simulink model "Model_simulink_dyskretny_impact_torque_NO_QUANTIZER"  (R2017a)
settings: Solver=ode45  StartTime=0.0  StopTime=Tend  FixedStep=Tp  RelTol=1e-3
values from neighbouring files (symbols this model uses):
  In = 130.7    [Skrypt_do_schematu.m]
  J = Js+Jmr    (= 5.82)    [Skrypt_do_schematu.m]
  K1 = Kw    [Skrypt_do_schematu.m]
  K2 = Kw*(Tp/TR-1)    [Skrypt_do_schematu.m]
  K3 = m/V    [Skrypt_do_schematu.m]
  K4 = (Tp-m)/V    [Skrypt_do_schematu.m]
  Kp = 0.15*Un    (= 66)    [Skrypt_do_schematu.m]
  Kt = 10/(1.2*wn)    (= 0.0548810148593)    [Skrypt_do_schematu.m]
  Lambda = 2    [Skrypt_do_schematu.m]
  Mn = psi * In    (= 350.156554572)    [Skrypt_do_schematu.m]
  psi = (Un-(Rt*In))/wn    (= 2.67908610996)    [Skrypt_do_schematu.m]
  Rt = 0.254    [Skrypt_do_schematu.m]
  T = Lt/Rt    (= 0.00641732283465)    [Skrypt_do_schematu.m]
  Tp = Beta/N    (= 0.002)    [Skrypt_do_schematu.m]
  Un = 440    [Skrypt_do_schematu.m]
  Uz0 = (Lambda*In)*((Y*B1)/(B1-Beta))    [Skrypt_do_schematu.m]
  wn = (2*pi*n)/60    (= 151.843644924)    [Skrypt_do_schematu.m]
  Y = 7.8/(2.5*In)    (= 0.0238714613619)    [Skrypt_do_schematu.m]
settings Model: Creator=user  LastModifiedBy=a
settings DataIOCC: LimitDataPoints=on  SaveFormat=Array  SignalLoggingSaveFormat=ModelDataLogs
settings OptimizationCC: BlockReduction=off  BooleanDataType=off  ExpressionDepthLimit=2147483647  LifeSpan=inf
settings DebuggingCC: SaveWithParameterizedLinksMsg=none  UnderspecifiedInitializationDetection=Classic  MergeDetectMultiDrivingBlocksExec=none  SignalResolutionControl=TryResolveAllWithWarning  MultiTaskDSMMsg=warning  MultiTaskCondExecSysMsg=none  StateNameClashWarn=warning  SFUnexpectedBacktrackingDiag=warning  SFNoUnconditionalDefaultTransitionDiag=warning  SFExecutionAtInitializationDiag=none
settings HardwareCC: ProdBitPerPointer=32  ProdBitPerSizeT=32  ProdBitPerPtrDiffT=32  ProdLargestAtomicFloat=None  ProdIntDivRoundTo=Undefined  ProdEndianess=Unspecified  ProdWordSize=32  ProdHWDeviceType=32-bit Generic  TargetUnknown=on
settings ModelReferenceCC: PropagateSignalLabelsOutOfModel=off
settings GRTTargetCC: TargetLangStandard=C89/C90 (ANSI)  GeneratePreprocessorConditionals=Disable all
settings ConfigComp: CovMetricSettings=dw  CovHtmlReporting=on  CovSaveCumulativeToWorkspaceVar=on  CovSaveSingleToWorkspaceVar=on  CovExternalEMLEnable=off

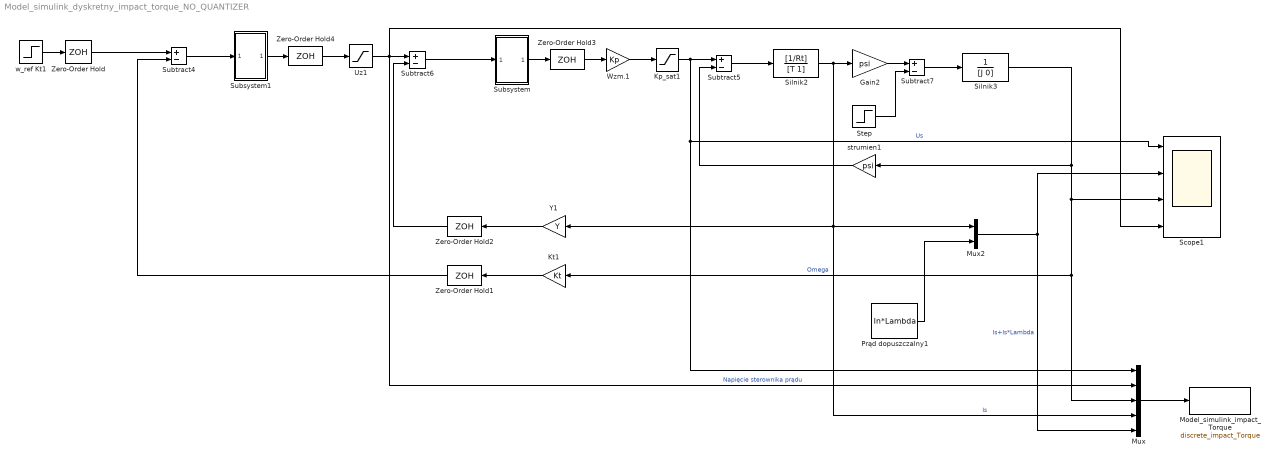
== system Model_simulink_dyskretny_impact_torque_NO_QUANTIZER ==
  Gain2 : Gain  Gain=psi
  Kp_sat1 : Saturate  UpperLimit=1.5*Un  LowerLimit=-1.5*Un
  Kt1 : Gain  Gain=Kt
  Model_simulink_impact_Torque : ToWorkspace  VariableName=discrete_impact_Torque  SaveFormat=Structure With Time  SampleTime=Tp
  Mux : Mux  Inputs=5
  Mux2 : Mux  Inputs=2
  Prąd dopuszczalny1 : Constant  Value=In*Lambda
  Scope1 : Scope  NumInputPorts=4
  Silnik2 : TransferFcn  Numerator=[1/Rt]  Denominator=[T 1]
  Silnik3 : TransferFcn  Numerator=1  Denominator=[J 0]
  Step : Step  Time=5  After=Mn  SampleTime=0
  Subsystem : Subsystem
  Subsystem1 : Subsystem
  Subtract{4..7} (4 alike) : Sum  Inputs=+-
  Uz1 : Saturate  UpperLimit=Uz0  LowerLimit=-Uz0  SampleTime=Tp
  Wzm.1 : Gain  Gain=Kp
  Y1 : Gain  Gain=Y
  Zero-Order Hold{,1..4} (5 alike) : ZeroOrderHold  SampleTime=Tp
  strumien1 : Gain  Gain=psi
  w_ref Kt1 : Step  Time=0  After=wn*Kt
  wires:
  w_ref Kt1/1 -> Zero-Order Hold/1
  Wzm.1/1 -> Kp_sat1/1
  Subtract5/1 -> Silnik2/1
  Silnik2/1 -> Mux/4, Y1/1, Mux2/1, Gain2/1  "Is"
  Gain2/1 -> Subtract7/1
  Subtract7/1 -> Silnik3/1
  strumien1/1 -> Subtract5/2
  Kp_sat1/1 -> Mux/1, Scope1/1, Subtract5/1  "Us"
  Y1/1 -> Zero-Order Hold2/1
  Mux2/1 -> Mux/5, Scope1/2  "Is+Is*Lambda"
  Prąd dopuszczalny1/1 -> Mux2/2
  Uz1/1 -> Mux/2, Scope1/4, Subtract6/1  "Napięcie sterownika prądu"
  Silnik3/1 -> Mux/3, Kt1/1, Scope1/3, strumien1/1  "Omega"
  Kt1/1 -> Zero-Order Hold1/1
  Step/1 -> Subtract7/2
  Mux/1 -> Model_simulink_impact_Torque/1
  Subtract6/1 -> Subsystem/1(In1)
  Subsystem1/1(Out1) -> Zero-Order Hold4/1
  Subtract4/1 -> Subsystem1/1(In1)
  Zero-Order Hold/1 -> Subtract4/1
  Zero-Order Hold2/1 -> Subtract6/2
  Zero-Order Hold1/1 -> Subtract4/2
  Zero-Order Hold3/1 -> Wzm.1/1
  Subsystem/1(Out1) -> Zero-Order Hold3/1
  Zero-Order Hold4/1 -> Uz1/1

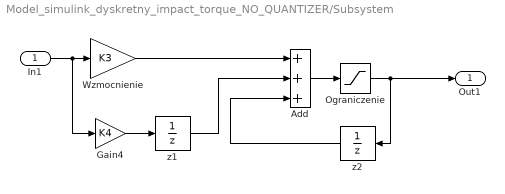
== system Model_simulink_dyskretny_impact_torque_NO_QUANTIZER/Subsystem ==
  In1 : Inport
  Add : Sum  Inputs=+++
  Gain4 : Gain  Gain=K4  SampleTime=Tp
  Ograniczenie : Saturate  UpperLimit=10  LowerLimit=-10
  Wzmocnienie : Gain  Gain=K3  SampleTime=Tp
  z1 : UnitDelay  SampleTime=Tp
  z2 : UnitDelay  SampleTime=Tp
  Out1 : Outport
  wires:
  In1/1 -> Gain4/1, Wzmocnienie/1
  Wzmocnienie/1 -> Add/1
  Gain4/1 -> z1/1
  z1/1 -> Add/2
  Add/1 -> Ograniczenie/1
  Ograniczenie/1 -> Out1/1, z2/1
  z2/1 -> Add/3

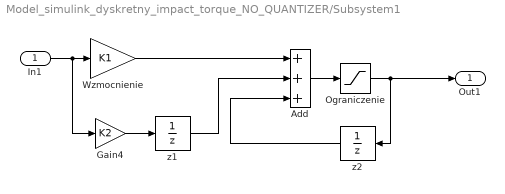
== system Model_simulink_dyskretny_impact_torque_NO_QUANTIZER/Subsystem1 ==
  In1 : Inport
  Add : Sum  Inputs=+++  SampleTime=Tp
  Gain4 : Gain  Gain=K2  SampleTime=Tp
  Ograniczenie : Saturate  UpperLimit=10  LowerLimit=-10
  Wzmocnienie : Gain  Gain=K1  SampleTime=Tp
  z1 : UnitDelay  SampleTime=Tp
  z2 : UnitDelay  SampleTime=Tp
  Out1 : Outport
  wires:
  In1/1 -> Gain4/1, Wzmocnienie/1
  Wzmocnienie/1 -> Add/1
  Gain4/1 -> z1/1
  z1/1 -> Add/2
  Add/1 -> Ograniczenie/1
  Ograniczenie/1 -> Out1/1, z2/1
  z2/1 -> Add/3
